simulink model "adrc"  (R2016a)
settings: Solver=ode3  StartTime=0.0  StopTime=50  FixedStep=0.01  RelTol=1e-3
libraries: simulink x3
settings Model: Creator=LZ  LastModifiedBy=LZ

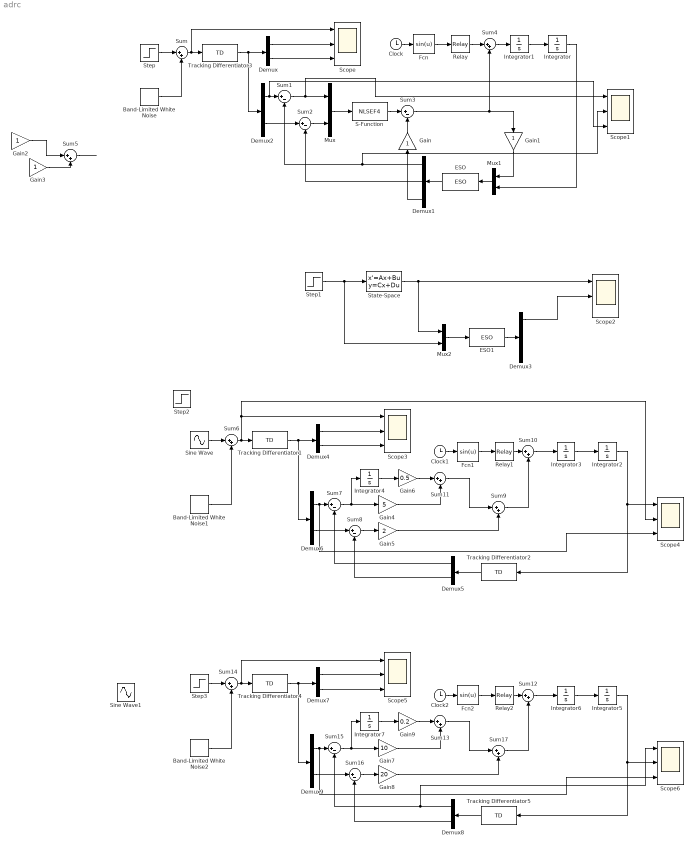
== system adrc ==
  Band-Limited White Noise : simulink/Sources/Band-Limited White Noise  Cov=0.0001  Ts=0.01  seed=[23341]
  Band-Limited White Noise1 : simulink/Sources/Band-Limited White Noise  Cov=0.0001  Ts=0.01  seed=[23341]
  Band-Limited White Noise2 : simulink/Sources/Band-Limited White Noise  Cov=0.0001  Ts=0.01  seed=[23341]
  Clock : Clock
  Clock1 : Clock
  Clock2 : Clock
  Demux{,2,4..9} (8 alike) : Demux  Outputs=2
  Demux1 : Demux  Outputs=3
  Demux3 : Demux  Outputs=3
  ESO : S-Function  FunctionName=ESO  Parameters=h, b0, beta, d  SFunctionDeploymentMode=off  EnableBusSupport=off  mask{h=2, b0=2, beta=[10, 100, 100], d=[0.5, 0.25]}
  ESO1 : S-Function  FunctionName=ESO  Parameters=h, b0, beta, d  SFunctionDeploymentMode=off  EnableBusSupport=off  mask{h=2, b0=2, beta=[100, 100, 1000], d=[0.5, 0.25]}
  Fcn : Fcn  Expr=sin(u)
  Fcn1 : Fcn  Expr=sin(u)
  Fcn2 : Fcn  Expr=sin(u)
  Gain{,1..3} (4 alike) : Gain
  Gain4 : Gain  Gain=5
  Gain5 : Gain  Gain=2
  Gain6 : Gain  Gain=0.5
  Gain7 : Gain  Gain=10
  Gain8 : Gain  Gain=20
  Gain9 : Gain  Gain=0.2
  Integrator{,1..7} (8 alike) : Integrator
  Mux : Mux  Inputs=2
  Mux1 : Mux  Inputs=2
  Mux2 : Mux  Inputs=2
  Relay : Relay
  Relay1 : Relay
  Relay2 : Relay
  S-Function : S-Function  FunctionName=NLSEF4  Parameters=c, r, h1  SFunctionDeploymentMode=off  EnableBusSupport=off  mask{c=2, r=1, h1=0.5}
  Scope{,1..6} (7 alike) : Scope  NumInputPorts=3
  Sine Wave : Sin  Amplitude=2  SampleTime=0
  Sine Wave1 : Sin  Amplitude=2  SampleTime=0
  State-Space : StateSpace  A=[0 1; 2 10]  B=[0; 2]  C=[1 0]  D=0  X0=0
  Step{,1..3} (4 alike) : Step  Time=3  After=10  SampleTime=0
  Sum{,5..6,9..14,17} (10 alike) : Sum  Inputs=|++
  Sum{1..3,7..8,15..16} (7 alike) : Sum  Inputs=|+-
  Sum4 : Sum  Inputs=|++  SaturateOnIntegerOverflow=on  InputSameDT=on  OutDataTypeStr=Inherit: Same as first input
  Tracking Differentiator1 : S-Function  FunctionName=TD  Parameters=r, h, n0  SFunctionDeploymentMode=off  EnableBusSupport=off  mask{r=30000, h=2, n0=20}
  Tracking Differentiator2 : S-Function  FunctionName=TD  Parameters=r, h, n0  SFunctionDeploymentMode=off  EnableBusSupport=off  mask{r=3000, h=2, n0=30}
  Tracking Differentiator3 : S-Function  FunctionName=TD  Parameters=r, h, n0  SFunctionDeploymentMode=off  EnableBusSupport=off  mask{r=30000, h=2, n0=20}
  Tracking Differentiator4 : S-Function  FunctionName=TD  Parameters=r, h, n0  SFunctionDeploymentMode=off  EnableBusSupport=off  mask{r=30000, h=2, n0=5}
  Tracking Differentiator5 : S-Function  FunctionName=TD  Parameters=r, h, n0  SFunctionDeploymentMode=off  EnableBusSupport=off  mask{r=3000, h=2, n0=30}
  wires:
  Step/1 -> Sum/1
  Sum/1 -> Tracking Differentiator3/1, Scope/1
  Tracking Differentiator3/1 -> Demux2/1, Demux/1
  Demux/1 -> Scope/2
  Demux/2 -> Scope/3
  Band-Limited White Noise/1 -> Sum/2
  ESO/1 -> Demux1/1
  Demux2/1 -> Scope1/3, Sum1/1
  Demux2/2 -> Sum2/1
  Gain/1 -> Sum3/2
  Sum3/1 -> Gain1/1, Sum4/2
  Mux1/1 -> ESO/1
  Gain1/1 -> Mux1/1
  Mux2/1 -> ESO1/1
  Step1/1 -> Mux2/2, State-Space/1
  State-Space/1 -> Mux2/1, Scope2/1
  ESO1/1 -> Demux3/1
  Demux3/1 -> Scope2/2
  Clock/1 -> Fcn/1
  Sum4/1 -> Integrator1/1
  Integrator1/1 -> Integrator/1
  Fcn/1 -> Relay/1
  Relay/1 -> Sum4/1
  Integrator/1 -> Mux1/2
  Mux/1 -> S-Function/1
  Sum1/1 -> Scope1/1, Mux/1
  Sum5/1 -> ?
  ? -> Gain3/1
  Gain3/1 -> Sum5/2
  Gain2/1 -> Sum5/1
  S-Function/1 -> Sum3/1
  Sum2/1 -> Mux/2
  Sum6/1 -> Scope4/2, Scope3/1, Tracking Differentiator1/1
  Tracking Differentiator1/1 -> Demux6/1, Demux4/1
  Demux4/1 -> Scope3/2
  Demux4/2 -> Scope3/3
  Band-Limited White Noise1/1 -> Sum6/2
  Demux6/1 -> Scope4/3, Sum7/1
  Demux6/2 -> Sum8/1
  Sum7/1 -> Integrator4/1, Gain4/1
  Sum11/1 -> Sum9/1
  Sum8/1 -> Gain5/1
  Integrator2/1 -> Tracking Differentiator2/1, Scope4/1
  Tracking Differentiator2/1 -> Demux5/1
  Demux5/1 -> Sum7/2
  Demux5/2 -> Sum8/2
  Integrator4/1 -> Gain6/1
  Gain4/1 -> Sum11/2
  Gain5/1 -> Sum9/2
  Integrator3/1 -> Integrator2/1
  Clock1/1 -> Fcn1/1
  Fcn1/1 -> Relay1/1
  Relay1/1 -> Sum10/1
  Sum9/1 -> Sum10/2
  Sum10/1 -> Integrator3/1
  Gain6/1 -> Sum11/1
  Sine Wave/1 -> Sum6/1
  Demux1/1 -> Scope1/2, Sum1/2
  Demux1/2 -> Sum2/2
  Demux1/3 -> Gain/1
  Sum14/1 -> Scope5/1, Tracking Differentiator4/1
  Tracking Differentiator4/1 -> Demux9/1, Demux7/1
  Demux7/1 -> Scope5/2
  Demux7/2 -> Scope5/3
  Demux9/1 -> Scope6/3, Sum15/1
  Demux9/2 -> Sum16/1
  Sum15/1 -> Integrator7/1, Gain7/1
  Sum13/1 -> Sum17/1
  Sum16/1 -> Gain8/1
  Integrator5/1 -> Tracking Differentiator5/1, Scope6/2
  Tracking Differentiator5/1 -> Demux8/1
  Demux8/1 -> Scope6/1, Sum15/2
  Demux8/2 -> Sum16/2
  Integrator7/1 -> Gain9/1
  Gain7/1 -> Sum13/2
  Gain8/1 -> Sum17/2
  Integrator6/1 -> Integrator5/1
  Clock2/1 -> Fcn2/1
  Fcn2/1 -> Relay2/1
  Relay2/1 -> Sum12/1
  Sum17/1 -> Sum12/2
  Sum12/1 -> Integrator6/1
  Gain9/1 -> Sum13/1
  Step3/1 -> Sum14/1
  Band-Limited White Noise2/1 -> Sum14/2
